simulink model "mech_robot_vr"  (Simulink 7.1)
settings: Solver=ode15s  StartTime=0.0  StopTime=1  RelTol=1e-3  AbsTol=1e-4
PreLoadFcn:
  | load mech_robot_images;mech_robot_data;
undefined symbols (not defined in the file or in its folder): Actuator, rad, s
libraries: mblibv1 x88
(part 2 of 4)

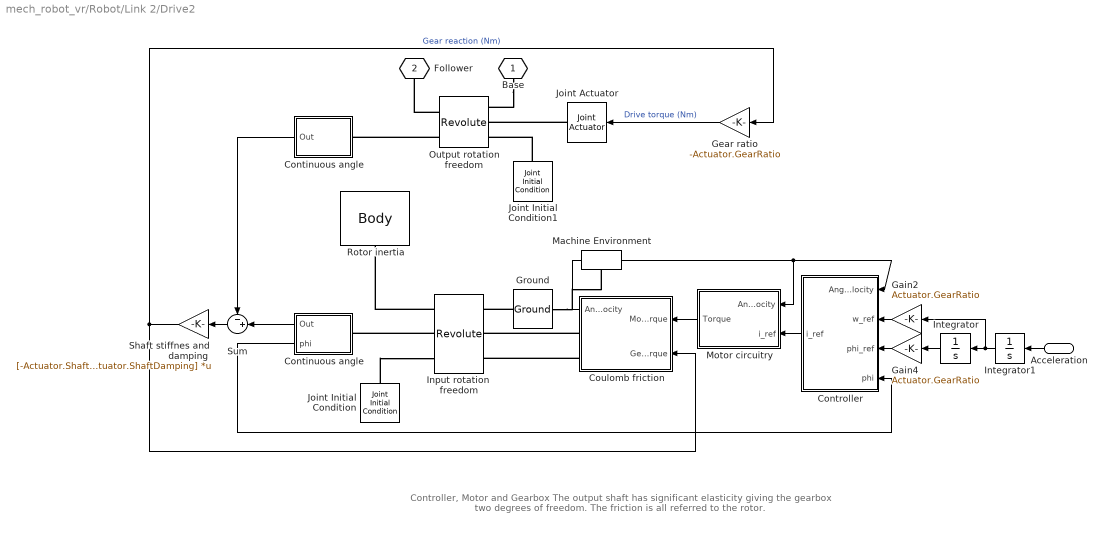
== system mech_robot_vr/Robot/Link 2/Drive2 ==
  note: Controller, Motor and Gearbox
      |
      | The output shaft has significant elasticity giving the gearbox two
      | degrees of freedom. The friction is all referred to the rotor.
  Acceleration : Inport  Orientation=left  OutDataType=sfix(16)  OutScaling=2^0
  Continuous angle : Subsystem  Orientation=left
  "Continuous angle " : Subsystem  Orientation=left
  Controller : Subsystem  Orientation=left
  Coulomb friction : Subsystem  Orientation=left  mask{peak=Actuator.PeakRatio, Rv1=Actuator.FrictionGain, Rv0=Actuator.FrictionConstant}
      mask prompts: peak "Peak ratio"; Rv1 "Friction gain (Nm.s/rad)"; Rv0 "Friction constant (Nm)"
      mask Display:
      | plot([-2 0 0 2],[-2 -1 1 2]);
      | plot([-5 5],[0 0]);
      | plot([0 0],[-5 5]);
      | plot([-0.02 -0.02],[-3 3]);
      | plot([-0.04 -0.04],[-3 3]);
      | plot([-0.06 -0.06],[-3 3]);
      | plot([-0.08 -0.08],[-3 3]);
      | plot([-0.1 -0.1],[-3 3]);
      | plot([0.02 0.02],[-3 3]);
      | plot([0.04 0.04],[-3 3]);
      | plot([0.06 0.06],[-3 3]);
      | plot([0.08 0.08],[-3 3]);
      | plot([0.1 0.1],[-3 3]);
      | plot([-2 0],[-2.03 -1.03]);
      | plot([-2 0],[-2.06 -1.06]);
      | plot([-2 0],[-2.09 -1.09]);
      | plot([-2 0],[-2.12 -1.21]);
      | plot([-2 0],[-1.97 -0.97]);
      | plot([-2 0],[-1.94 -0.94]);
      | plot([-2 0],[-1.91 -0.91]);
      | plot([-2 0],[-1.88 -0.88]);
      | 
      | plot([2 0],[2.03 1.03]);
      | plot([2 0],[2.06 1.06]);
      | plot([2 0],[2.09 1.09]);
      | plot([2 0],[2.12 1.21]);
      | plot([2 0],[1.97 0.97]);
      | plot([2 0],[1.94 0.94]);
      | plot([2 0],[1.91 0.91]);
      | plot([2 0],[1.88 0.88]);
  Gain2 : Gain  Orientation=left  Gain=Actuator.GearRatio  ParameterDataType=sfix(16)  ParameterScaling=2^0  OutDataType=sfix(16)  OutScaling=2^0  SaturateOnIntegerOverflow=on  OutDataTypeStr=Inherit: Same as input  ParamDataTypeStr=Inherit: Same as input
  Gain4 : Gain  Orientation=left  Gain=Actuator.GearRatio  ParameterDataType=sfix(16)  ParameterScaling=2^0  OutDataType=sfix(16)  OutScaling=2^0  SaturateOnIntegerOverflow=on  OutDataTypeStr=Inherit: Same as input  ParamDataTypeStr=Inherit: Same as input
  Gear ratio : Gain  Orientation=left  Gain=-Actuator.GearRatio  ParameterDataType=sfix(16)  ParameterScaling=2^0  OutDataType=sfix(16)  OutScaling=2^0  SaturateOnIntegerOverflow=on  OutDataTypeStr=Inherit: Same as input  ParamDataTypeStr=Inherit: Same as input
  Ground : mblibv1/Bodies/Ground  Orientation=left  DialogController=MECH.DynMechDlgSource  SystemSampleTime=-1  LeftPortType=env  RightPortType=workingframe  PhysicalDomain=Mechanical  DialogClass=GroundBlock  CoordPosition=[0 0 0]  CoordPositionUnits=m  StateVectorMgrId=-1  MachineId=[0 0]  ShowEnvPort=on
  Input rotation  freedom : mblibv1/Joints/Revolute  Tag=Factory generic  Description=Mechanical Blockset  Orientation=left  DialogController=MECH.DynMechDlgSource  PhysicalDomain=mechanical  SubClassName=Unknown  LeftPortType=blob  RightPortType=blob  LConnTagsString=__newl0|SA1|SA2  RConnTagsString=__newr0|SA1|SA2  NumSAPorts=4  CutJoint=off  MarkAsCut=off  Primitives=revolute  PrimitiveProps=R1$WORLD$Actuator.Axis$revolute  DialogClass=JointBlock  R1Axis=Actuator.Axis
  Integrator : Integrator  Orientation=left  InitialCondition=q0  ZeroCross=off
  Integrator1 : Integrator  Orientation=left  ZeroCross=off
  Joint Actuator : mblibv1/Sensors &  Actuators/Joint Actuator  Orientation=left  DialogController=MECH.DynMechDlgSource  SystemSampleTime=-1  PhysicalDomain=Mechanical  PortType=blob  ActuationStyle=Force  AngleUnits=deg  ArcVelocityUnits=deg/s  ArcAccelerationUnits=deg/s^2  CoordPositionUnits=m  VelocityUnits=m/s  AccelerationUnits=m/s^2  ForceUnits=N  TorqueUnits=N-m  ActiveIO=on  Width=1  DialogClass=MechanicalActuatorBlock  Primitive=R1  ReferenceFrame=Absolute (INERTIAL)
  Joint Initial Condition : mblibv1/Sensors &  Actuators/Joint Initial Condition  Orientation=up  DialogController=MECH.DynMechDlgSource  SystemSampleTime=-1  PhysicalDomain=Mechanical  DialogClass=InitialConditionBlock  Primitive=R1  CoordPosition=q0*Actuator.GearRatio  Velocity=0.0  AngleUnits=rad  ArcVelocityUnits=deg/s  CoordPositionUnits=m  VelocityUnits=m/s  InitialConditions=P1$false$0$m$rad$0$m/s$rad/s#P2$false$0$m$rad$0$m/s$rad/s#P3$false$0$m$rad$0$m/s$rad/s#R1$true$q0*Actuator.GearRatio$m$rad$0.0$m/s$deg/s#R2$false$0$m$rad$0$m/s$rad/s#R3$false$0$m$rad$0$m/s$rad/s#S$false$0$m$rad$0$m/s$rad/s  P1PIC=0  P1VIC=0  P2PIC=0  P2VIC=0  P3PIC=0  P3VIC=0  R1PIC=q0*Actuator.GearRatio  R1VIC=0.0  R2PIC=0  R2VIC=0  R3PIC=0  R3VIC=0  SPIC=0  SVIC=0
  Joint Initial Condition1 : mblibv1/Sensors &  Actuators/Joint Initial Condition  Orientation=up  DialogController=MECH.DynMechDlgSource  SystemSampleTime=-1  PhysicalDomain=Mechanical  DialogClass=InitialConditionBlock  Primitive=R1  CoordPosition=q0  Velocity=0.0  AngleUnits=rad  ArcVelocityUnits=deg/s  CoordPositionUnits=m  VelocityUnits=m/s  InitialConditions=P1$false$0$m$rad$0$m/s$rad/s#P2$false$0$m$rad$0$m/s$rad/s#P3$false$0$m$rad$0$m/s$rad/s#R1$true$q0$m$rad$0.0$m/s$deg/s#R2$false$0$m$rad$0$m/s$rad/s#R3$false$0$m$rad$0$m/s$rad/s#S$false$0$m$rad$0$m/s$rad/s  P1PIC=0  P1VIC=0  P2PIC=0  P2VIC=0  P3PIC=0  P3VIC=0  R1PIC=q0  R1VIC=0.0  R2PIC=0  R2VIC=0  R3PIC=0  R3VIC=0  SPIC=0  SVIC=0
  Machine Environment : mblibv1/Bodies/Machine Environment  Tag=Factory ground  Orientation=down  DialogController=MECH.DialogSource  SystemSampleTime=-1  PortType=env  PhysicalDomain=Mechanical  DialogTemplateClass=MECH.MachineEnvironment  SyncWhenCopied=off  Gravity=[0 -9.81 0]  GravityUnits=m/s^2  GravityAsSignal=off  Dimensionality=3D Only  AnalysisType=Forward dynamics  LinearAssemblyTolerance=1e-3  LinearAssemblyToleranceUnits=m  AngularAssemblyTolerance=1e-3  AngularAssemblyToleranceUnits=rad  ConstraintSolverType=Stabilizing  ConstraintRelTolerance=1e-4  ConstraintAbsTolerance=1e-4  UseRobustSingularityHandling=off  RedundancyAnalysisToleranceType=Automatically select tolerance  RedundancyAnalysisTolerance=1e-14  StatePerturbationType=Fixed  PerturbationSize=1e-5  VisualizeMachine=on
  Motor circuitry : Subsystem  Orientation=left  mask{Ri=10, Ra=250, Rd1=100, Rd2=100, Rd3=100, Rd4=100, Rp1=200, Rp2=50, k=Actuator.MotorGain, d=Actuator.MotorDamping, w=Actuator.MotorConstant}
      mask prompts: Ri "Ri (Ohms)"; Ra "Ra (Ohms)"; Rd1 "Rd1 (Ohms)"; Rd2 "Rd2 (Ohms)"; Rd3 "Rd3 (Ohms)"; Rd4 "Rd4 (Ohms)"; Rp1 "Rp1 (Ohms)"; Rp2 "Rp2 (Ohms)"; k "Motor gain (Nm/A)"; d "Motor damping"; w "Motor time constant"
      mask Display: plot(-140,-140,140,140,2*[-30,-30,0,-30,-30,-55]+25,(2*[20,0,20,41,20,20]+8),[0,0]+25,(2*[0,40]+8),2*[37.5,0]+25,(2*[20,20]+8),2*[10,10,0]+25,(1*[-15,6,20]+12),1*[-65,-65,-20,-20,40,40,85,85,85,40,40,-20,-20],1*[48,-20,-20,-10,-10,-20,-20,48,-20,-20,-30,-30,-20])
  Output rotation freedom : mblibv1/Joints/Revolute  Tag=Factory generic  Description=Mechanical Blockset  Orientation=left  DialogController=MECH.DynMechDlgSource  PhysicalDomain=mechanical  SubClassName=Unknown  LeftPortType=blob  RightPortType=blob  LConnTagsString=__newl0|SA1|SA2  RConnTagsString=__newr0|SA1  NumSAPorts=3  CutJoint=off  MarkAsCut=off  Primitives=revolute  PrimitiveProps=R1$WORLD$Actuator.Axis$revolute  DialogClass=JointBlock  R1Axis=Actuator.Axis
  Rotor inertia : mblibv1/Bodies/Body  Tag=Factory generic  Description=Mechanical Blockset  Orientation=up  DialogController=MECH.DynMechDlgSource  PhysicalDomain=mechanical  SubClassName=Unknown  LeftPortType=workingframe  RightPortType=workingframe  LConnTagsString=CS1  DialogClass=MechanicalBodyBlock  Mass=0.5  MassUnits=kg  InertiaUnits=kg*m^2  Inertia=Actuator.MotorInertia*eye(3)  Shape=Cylinder  ShapeDims=[1 1]  ShapeUnits=m  ShapeUse=false  Density=1  DensityUnits=kg/m^3  DensityUse=false  GraphicsMode=1  BodyColor=[0.5 0.5 0.5]  GraphicsObj=[]  AttachedToCS=1  CG=Left$CG$[0 0 0]$CS1$CS1$m$[0 0 0]$Euler X-Y-Z$deg$WORLD$false  WorkingFrames=Left$CS1$[0 0 0]$ADJOINING$ADJOINING$m$[0 0 0]$Euler X-Y-Z$deg$WORLD$true  CGPos=[0 0 0]  CGRot=[0 0 0]  CS0Pos=[]  CS0Rot=[]  CS1Pos=[0 0 0]  CS1Rot=[0 0 0]  CS2Pos=[]  CS2Rot=[]  CS3Pos=[]  CS3Rot=[]  CS4Pos=[]  CS4Rot=[]  CS5Pos=[]  CS5Rot=[]  CS6Pos=[]  CS6Rot=[]  CS7Pos=[]  CS7Rot=[]  CS8Pos=[]  CS8Rot=[]  CS9Pos=[]  CS9Rot=[]  CS10Pos=[]  CS10Rot=[]  CS11Pos=[]  CS11Rot=[]  CS12Pos=[]  CS12Rot=[]  CS13Pos=[]  CS13Rot=[]  CS14Pos=[]  CS14Rot=[]  CS15Pos=[]  CS15Rot=[]  CS16Pos=[]  CS16Rot=[]  CS17Pos=[]  CS17Rot=[]  CS18Pos=[]  CS18Rot=[]  CS19Pos=[]  CS19Rot=[]  CS20Pos=[]  CS20Rot=[]
  Shaft stiffnes and damping : Gain  Orientation=left  Gain=[-Actuator.ShaftStiffness -Actuator.ShaftDamping]  Multiplication=Matrix(K*u)  ParameterDataType=sfix(16)  ParameterScaling=2^0  OutDataType=sfix(16)  OutScaling=2^0  SaturateOnIntegerOverflow=on  OutDataTypeStr=Inherit: Same as input  ParamDataTypeStr=Inherit: Same as input
  Sum : Sum  Orientation=left  Inputs=-+|  OutDataType=sfix(16)  OutScaling=2^0  SaturateOnIntegerOverflow=on  InputSameDT=on  OutDataTypeStr=Inherit: Same as first input
  Base : PMIOPort  Tag=PMCPort  Orientation=down  Port=1  Side=Left
  Follower : PMIOPort  Tag=PMCPort  Orientation=down  Port=2  Side=Right
  wires:
  Coulomb friction/1(Angular velocity) -> Controller/1(Angular velocity), Motor circuitry/1(Angular velocity)
  Gear ratio/1 -> Joint Actuator/1  "Drive torque (Nm)"
  Integrator/1 -> Gain4/1
  Acceleration/1 -> Integrator1/1
  "Continuous angle "/1("Out ") -> Sum/1
  Gain2/1 -> Controller/2(w_ref)
  Gain4/1 -> Controller/3(phi_ref)
  Motor circuitry/1(Torque) -> Coulomb friction/1(Motor torque)
  Sum/1 -> Shaft stiffnes and damping/1
  Continuous angle/1(Out) -> Sum/2
  Continuous angle/2(phi) -> Controller/4(phi)
  Shaft stiffnes and damping/1 -> Gear ratio/1, Coulomb friction/2(Gear torque)  "Gear reaction (Nm)"
  Integrator1/1 -> Integrator/1, Gain2/1
  Controller/1(i_ref) -> Motor circuitry/2(i_ref)
  connections:
  Base/RConn1 -- Output rotation freedom/LConn1
  Output rotation freedom/RConn1 -- Follower/RConn1
  Output rotation freedom/RConn2 -- "Continuous angle "/LConn1
  Coulomb friction/RConn1 -- Input rotation  freedom/LConn2
  Coulomb friction/RConn2 -- Input rotation  freedom/LConn3
  Input rotation  freedom/RConn1 -- Rotor inertia/LConn1
  Input rotation  freedom/RConn2 -- Continuous angle/LConn1
  Ground/RConn1 -- Input rotation  freedom/LConn1
  Joint Initial Condition1/RConn1 -- Output rotation freedom/LConn3
  Joint Actuator/RConn1 -- Output rotation freedom/LConn2
  Joint Initial Condition/RConn1 -- Input rotation  freedom/RConn3
  Ground/LConn1 -- Machine Environment/RConn1

== system mech_robot_vr/Robot/Link 2/Subsystem ==
  Clock1 : Clock
      settings: Decimation=10
  Trajectory 2 : Lookup  InputValues="[0    0.1000    0.1000    1.1000    1.1000    1.2000    1.2000    1.3000]"  Table="[-15   -15     0     0    15    15     0     0]"  OutDataType=sfix(16)  OutScaling=2^0  SaturateOnIntegerOverflow=on
  Acceleration2 : Outport  OutDataType=sfix(16)  OutScaling=2^0
  wires:
  Clock1/1 -> Trajectory 2/1
  Trajectory 2/1 -> Acceleration2/1

== system mech_robot_vr/Robot/Link3/Acceleration3 ==
  Clock5 : Clock
      settings: Decimation=10
  Trajectory 3 : Lookup  InputValues="[0    0.1500    0.1500    0.6000    0.6000    0.9000    0.9000    1.2000    1.2000    1.3000]"  Table="[30.0000   30.0000  -21.5600  -21.5600         0         0   17.3300   17.3300         0         0]"  OutDataType=sfix(16)  OutScaling=2^0  SaturateOnIntegerOverflow=on
  Acceleration3 : Outport  OutDataType=sfix(16)  OutScaling=2^0
  wires:
  Clock5/1 -> Trajectory 3/1
  Trajectory 3/1 -> Acceleration3/1

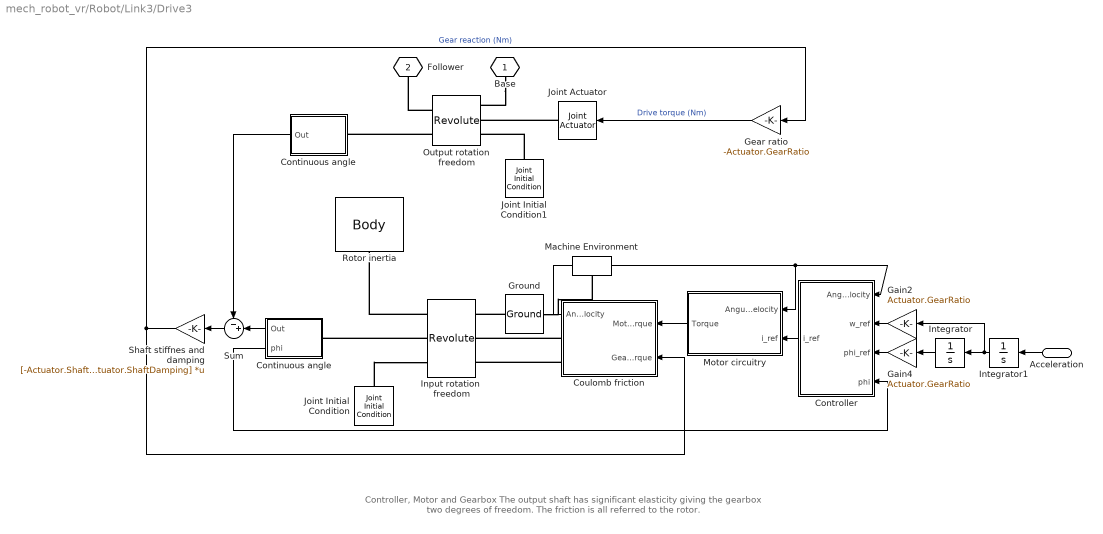
== system mech_robot_vr/Robot/Link3/Drive3 ==
  note: Controller, Motor and Gearbox
      |
      | The output shaft has significant elasticity giving the gearbox two
      | degrees of freedom. The friction is all referred to the rotor.
  Acceleration : Inport  Orientation=left  OutDataType=sfix(16)  OutScaling=2^0
  Continuous angle : Subsystem  Orientation=left
  "Continuous angle " : Subsystem  Orientation=left
  Controller : Subsystem  Orientation=left
  Coulomb friction : Subsystem  Orientation=left  mask{peak=Actuator.PeakRatio, Rv1=Actuator.FrictionGain, Rv0=Actuator.FrictionConstant}
      mask prompts: peak "Peak ratio"; Rv1 "Friction gain (Nm.s/rad)"; Rv0 "Friction constant (Nm)"
      mask Display:
      | plot([-2 0 0 2],[-2 -1 1 2]);
      | plot([-5 5],[0 0]);
      | plot([0 0],[-5 5]);
      | plot([-0.02 -0.02],[-3 3]);
      | plot([-0.04 -0.04],[-3 3]);
      | plot([-0.06 -0.06],[-3 3]);
      | plot([-0.08 -0.08],[-3 3]);
      | plot([-0.1 -0.1],[-3 3]);
      | plot([0.02 0.02],[-3 3]);
      | plot([0.04 0.04],[-3 3]);
      | plot([0.06 0.06],[-3 3]);
      | plot([0.08 0.08],[-3 3]);
      | plot([0.1 0.1],[-3 3]);
      | plot([-2 0],[-2.03 -1.03]);
      | plot([-2 0],[-2.06 -1.06]);
      | plot([-2 0],[-2.09 -1.09]);
      | plot([-2 0],[-2.12 -1.21]);
      | plot([-2 0],[-1.97 -0.97]);
      | plot([-2 0],[-1.94 -0.94]);
      | plot([-2 0],[-1.91 -0.91]);
      | plot([-2 0],[-1.88 -0.88]);
      | 
      | plot([2 0],[2.03 1.03]);
      | plot([2 0],[2.06 1.06]);
      | plot([2 0],[2.09 1.09]);
      | plot([2 0],[2.12 1.21]);
      | plot([2 0],[1.97 0.97]);
      | plot([2 0],[1.94 0.94]);
      | plot([2 0],[1.91 0.91]);
      | plot([2 0],[1.88 0.88]);
  Gain2 : Gain  Orientation=left  Gain=Actuator.GearRatio  ParameterDataType=sfix(16)  ParameterScaling=2^0  OutDataType=sfix(16)  OutScaling=2^0  SaturateOnIntegerOverflow=on  OutDataTypeStr=Inherit: Same as input  ParamDataTypeStr=Inherit: Same as input
  Gain4 : Gain  Orientation=left  Gain=Actuator.GearRatio  ParameterDataType=sfix(16)  ParameterScaling=2^0  OutDataType=sfix(16)  OutScaling=2^0  SaturateOnIntegerOverflow=on  OutDataTypeStr=Inherit: Same as input  ParamDataTypeStr=Inherit: Same as input
  Gear ratio : Gain  Orientation=left  Gain=-Actuator.GearRatio  ParameterDataType=sfix(16)  ParameterScaling=2^0  OutDataType=sfix(16)  OutScaling=2^0  SaturateOnIntegerOverflow=on  OutDataTypeStr=Inherit: Same as input  ParamDataTypeStr=Inherit: Same as input
  Ground : mblibv1/Bodies/Ground  Orientation=left  DialogController=MECH.DynMechDlgSource  SystemSampleTime=-1  LeftPortType=env  RightPortType=workingframe  PhysicalDomain=Mechanical  DialogClass=GroundBlock  CoordPosition=[0 0 0]  CoordPositionUnits=m  StateVectorMgrId=-1  MachineId=[0 0]  ShowEnvPort=on
  Input rotation  freedom : mblibv1/Joints/Revolute  Tag=Factory generic  Description=Mechanical Blockset  Orientation=left  DialogController=MECH.DynMechDlgSource  PhysicalDomain=mechanical  SubClassName=Unknown  LeftPortType=blob  RightPortType=blob  LConnTagsString=__newl0|SA1|SA2  RConnTagsString=__newr0|SA1|SA2  NumSAPorts=4  CutJoint=off  MarkAsCut=off  Primitives=revolute  PrimitiveProps=R1$WORLD$Actuator.Axis$revolute  DialogClass=JointBlock  R1Axis=Actuator.Axis
  Integrator : Integrator  Orientation=left  InitialCondition=q0  ZeroCross=off
  Integrator1 : Integrator  Orientation=left  ZeroCross=off
  Joint Actuator : mblibv1/Sensors &  Actuators/Joint Actuator  Orientation=left  DialogController=MECH.DynMechDlgSource  SystemSampleTime=-1  PhysicalDomain=Mechanical  PortType=blob  ActuationStyle=Force  AngleUnits=deg  ArcVelocityUnits=deg/s  ArcAccelerationUnits=deg/s^2  CoordPositionUnits=m  VelocityUnits=m/s  AccelerationUnits=m/s^2  ForceUnits=N  TorqueUnits=N-m  ActiveIO=on  Width=1  DialogClass=MechanicalActuatorBlock  Primitive=R1  ReferenceFrame=Absolute (INERTIAL)
  Joint Initial Condition : mblibv1/Sensors &  Actuators/Joint Initial Condition  Orientation=up  DialogController=MECH.DynMechDlgSource  SystemSampleTime=-1  PhysicalDomain=Mechanical  DialogClass=InitialConditionBlock  Primitive=R1  CoordPosition=q0*Actuator.GearRatio  Velocity=0.0  AngleUnits=rad  ArcVelocityUnits=deg/s  CoordPositionUnits=m  VelocityUnits=m/s  InitialConditions=P1$false$0$m$rad$0$m/s$rad/s#P2$false$0$m$rad$0$m/s$rad/s#P3$false$0$m$rad$0$m/s$rad/s#R1$true$q0*Actuator.GearRatio$m$rad$0.0$m/s$deg/s#R2$false$0$m$rad$0$m/s$rad/s#R3$false$0$m$rad$0$m/s$rad/s#S$false$0$m$rad$0$m/s$rad/s  P1PIC=0  P1VIC=0  P2PIC=0  P2VIC=0  P3PIC=0  P3VIC=0  R1PIC=q0*Actuator.GearRatio  R1VIC=0.0  R2PIC=0  R2VIC=0  R3PIC=0  R3VIC=0  SPIC=0  SVIC=0
  Joint Initial Condition1 : mblibv1/Sensors &  Actuators/Joint Initial Condition  Orientation=up  DialogController=MECH.DynMechDlgSource  SystemSampleTime=-1  PhysicalDomain=Mechanical  DialogClass=InitialConditionBlock  Primitive=R1  CoordPosition=q0  Velocity=0.0  AngleUnits=rad  ArcVelocityUnits=deg/s  CoordPositionUnits=m  VelocityUnits=m/s  InitialConditions=P1$false$0$m$rad$0$m/s$rad/s#P2$false$0$m$rad$0$m/s$rad/s#P3$false$0$m$rad$0$m/s$rad/s#R1$true$q0$m$rad$0.0$m/s$deg/s#R2$false$0$m$rad$0$m/s$rad/s#R3$false$0$m$rad$0$m/s$rad/s#S$false$0$m$rad$0$m/s$rad/s  P1PIC=0  P1VIC=0  P2PIC=0  P2VIC=0  P3PIC=0  P3VIC=0  R1PIC=q0  R1VIC=0.0  R2PIC=0  R2VIC=0  R3PIC=0  R3VIC=0  SPIC=0  SVIC=0
  Machine Environment : mblibv1/Bodies/Machine Environment  Tag=Factory ground  Orientation=down  DialogController=MECH.DialogSource  SystemSampleTime=-1  PortType=env  PhysicalDomain=Mechanical  DialogTemplateClass=MECH.MachineEnvironment  SyncWhenCopied=off  Gravity=[0 -9.81 0]  GravityUnits=m/s^2  GravityAsSignal=off  Dimensionality=3D Only  AnalysisType=Forward dynamics  LinearAssemblyTolerance=1e-3  LinearAssemblyToleranceUnits=m  AngularAssemblyTolerance=1e-3  AngularAssemblyToleranceUnits=rad  ConstraintSolverType=Stabilizing  ConstraintRelTolerance=1e-4  ConstraintAbsTolerance=1e-4  UseRobustSingularityHandling=off  RedundancyAnalysisToleranceType=Automatically select tolerance  RedundancyAnalysisTolerance=1e-14  StatePerturbationType=Fixed  PerturbationSize=1e-5  VisualizeMachine=on
  Motor circuitry : Subsystem  Orientation=left  mask{Ri=10, Ra=250, Rd1=100, Rd2=100, Rd3=100, Rd4=100, Rp1=200, Rp2=50, k=Actuator.MotorGain, d=Actuator.MotorDamping, w=Actuator.MotorConstant}
      mask prompts: Ri "Ri (Ohms)"; Ra "Ra (Ohms)"; Rd1 "Rd1 (Ohms)"; Rd2 "Rd2 (Ohms)"; Rd3 "Rd3 (Ohms)"; Rd4 "Rd4 (Ohms)"; Rp1 "Rp1 (Ohms)"; Rp2 "Rp2 (Ohms)"; k "Motor gain (Nm/A)"; d "Motor damping"; w "Motor time constant"
      mask Display: plot(-140,-140,140,140,2*[-30,-30,0,-30,-30,-55]+25,(2*[20,0,20,41,20,20]+8),[0,0]+25,(2*[0,40]+8),2*[37.5,0]+25,(2*[20,20]+8),2*[10,10,0]+25,(1*[-15,6,20]+12),1*[-65,-65,-20,-20,40,40,85,85,85,40,40,-20,-20],1*[48,-20,-20,-10,-10,-20,-20,48,-20,-20,-30,-30,-20])
  Output rotation freedom : mblibv1/Joints/Revolute  Tag=Factory generic  Description=Mechanical Blockset  Orientation=left  DialogController=MECH.DynMechDlgSource  PhysicalDomain=mechanical  SubClassName=Unknown  LeftPortType=blob  RightPortType=blob  LConnTagsString=__newl0|SA1|SA2  RConnTagsString=__newr0|SA1  NumSAPorts=3  CutJoint=off  MarkAsCut=off  Primitives=revolute  PrimitiveProps=R1$WORLD$Actuator.Axis$revolute  DialogClass=JointBlock  R1Axis=Actuator.Axis
  Rotor inertia : mblibv1/Bodies/Body  Tag=Factory generic  Description=Mechanical Blockset  Orientation=up  DialogController=MECH.DynMechDlgSource  PhysicalDomain=mechanical  SubClassName=Unknown  LeftPortType=workingframe  RightPortType=workingframe  LConnTagsString=CS1  DialogClass=MechanicalBodyBlock  Mass=0.5  MassUnits=kg  InertiaUnits=kg*m^2  Inertia=Actuator.MotorInertia*eye(3)  Shape=Cylinder  ShapeDims=[1 1]  ShapeUnits=m  ShapeUse=false  Density=1  DensityUnits=kg/m^3  DensityUse=false  GraphicsMode=1  BodyColor=[0.5 0.5 0.5]  GraphicsObj=[]  AttachedToCS=1  CG=Left$CG$[0 0 0]$CS1$CS1$m$[0 0 0]$Euler X-Y-Z$deg$WORLD$false  WorkingFrames=Left$CS1$[0 0 0]$ADJOINING$ADJOINING$m$[0 0 0]$Euler X-Y-Z$deg$WORLD$true  CGPos=[0 0 0]  CGRot=[0 0 0]  CS0Pos=[]  CS0Rot=[]  CS1Pos=[0 0 0]  CS1Rot=[0 0 0]  CS2Pos=[]  CS2Rot=[]  CS3Pos=[]  CS3Rot=[]  CS4Pos=[]  CS4Rot=[]  CS5Pos=[]  CS5Rot=[]  CS6Pos=[]  CS6Rot=[]  CS7Pos=[]  CS7Rot=[]  CS8Pos=[]  CS8Rot=[]  CS9Pos=[]  CS9Rot=[]  CS10Pos=[]  CS10Rot=[]  CS11Pos=[]  CS11Rot=[]  CS12Pos=[]  CS12Rot=[]  CS13Pos=[]  CS13Rot=[]  CS14Pos=[]  CS14Rot=[]  CS15Pos=[]  CS15Rot=[]  CS16Pos=[]  CS16Rot=[]  CS17Pos=[]  CS17Rot=[]  CS18Pos=[]  CS18Rot=[]  CS19Pos=[]  CS19Rot=[]  CS20Pos=[]  CS20Rot=[]
  Shaft stiffnes and damping : Gain  Orientation=left  Gain=[-Actuator.ShaftStiffness -Actuator.ShaftDamping]  Multiplication=Matrix(K*u)  ParameterDataType=sfix(16)  ParameterScaling=2^0  OutDataType=sfix(16)  OutScaling=2^0  SaturateOnIntegerOverflow=on  OutDataTypeStr=Inherit: Same as input  ParamDataTypeStr=Inherit: Same as input
  Sum : Sum  Orientation=left  Inputs=-+|  OutDataType=sfix(16)  OutScaling=2^0  SaturateOnIntegerOverflow=on  InputSameDT=on  OutDataTypeStr=Inherit: Same as first input
  Base : PMIOPort  Tag=PMCPort  Orientation=down  Port=1  Side=Left
  Follower : PMIOPort  Tag=PMCPort  Orientation=down  Port=2  Side=Right
  wires:
  Coulomb friction/1(Angular velocity) -> Controller/1(Angular velocity), Motor circuitry/1(Angular velocity)
  Gear ratio/1 -> Joint Actuator/1  "Drive torque (Nm)"
  Integrator/1 -> Gain4/1
  Acceleration/1 -> Integrator1/1
  "Continuous angle "/1("Out ") -> Sum/1
  Gain2/1 -> Controller/2(w_ref)
  Gain4/1 -> Controller/3(phi_ref)
  Controller/1(i_ref) -> Motor circuitry/2(i_ref)
  Motor circuitry/1(Torque) -> Coulomb friction/1(Motor torque)
  Sum/1 -> Shaft stiffnes and damping/1
  Continuous angle/1(Out) -> Sum/2
  Continuous angle/2(phi) -> Controller/4(phi)
  Integrator1/1 -> Integrator/1, Gain2/1
  Shaft stiffnes and damping/1 -> Gear ratio/1, Coulomb friction/2(Gear torque)  "Gear reaction (Nm)"
  connections:
  Base/RConn1 -- Output rotation freedom/LConn1
  Output rotation freedom/RConn1 -- Follower/RConn1
  Output rotation freedom/RConn2 -- "Continuous angle "/LConn1
  Coulomb friction/RConn1 -- Input rotation  freedom/LConn2
  Coulomb friction/RConn2 -- Input rotation  freedom/LConn3
  Input rotation  freedom/RConn1 -- Rotor inertia/LConn1
  Input rotation  freedom/RConn2 -- Continuous angle/LConn1
  Ground/RConn1 -- Input rotation  freedom/LConn1
  Joint Initial Condition1/RConn1 -- Output rotation freedom/LConn3
  Joint Actuator/RConn1 -- Output rotation freedom/LConn2
  Joint Initial Condition/RConn1 -- Input rotation  freedom/RConn3
  Ground/LConn1 -- Machine Environment/RConn1

== system mech_robot_vr/Robot/Link4/Drive4 ==
  note: Controller, motor and ideal gear
      | No elasticity is modelled in this gear. All friction is referred
      | to the rotor.
  Acceleration : Inport  Orientation=left  OutDataType=sfix(16)  OutScaling=2^0
  Continuous angle : Subsystem
  Controller : Subsystem  Orientation=left
  Coulomb friction : Subsystem  Orientation=left  mask{peak=Actuator.PeakRatio, Rv1=Actuator.FrictionGain, Rv0=Actuator.FrictionConstant}
      mask prompts: peak "Peak ratio"; Rv1 "Friction gain (Nm.s/rad)"; Rv0 "Friction constant (Nm)"
      mask Display:
      | plot([-2 0 0 2],[-2 -1 1 2]);
      | plot([-5 5],[0 0]);
      | plot([0 0],[-5 5]);
      | plot([-0.02 -0.02],[-3 3]);
      | plot([-0.04 -0.04],[-3 3]);
      | plot([-0.06 -0.06],[-3 3]);
      | plot([-0.08 -0.08],[-3 3]);
      | plot([-0.1 -0.1],[-3 3]);
      | plot([0.02 0.02],[-3 3]);
      | plot([0.04 0.04],[-3 3]);
      | plot([0.06 0.06],[-3 3]);
      | plot([0.08 0.08],[-3 3]);
      | plot([0.1 0.1],[-3 3]);
      | plot([-2 0],[-2.03 -1.03]);
      | plot([-2 0],[-2.06 -1.06]);
      | plot([-2 0],[-2.09 -1.09]);
      | plot([-2 0],[-2.12 -1.21]);
      | plot([-2 0],[-1.97 -0.97]);
      | plot([-2 0],[-1.94 -0.94]);
      | plot([-2 0],[-1.91 -0.91]);
      | plot([-2 0],[-1.88 -0.88]);
      | 
      | plot([2 0],[2.03 1.03]);
      | plot([2 0],[2.06 1.06]);
      | plot([2 0],[2.09 1.09]);
      | plot([2 0],[2.12 1.21]);
      | plot([2 0],[1.97 0.97]);
      | plot([2 0],[1.94 0.94]);
      | plot([2 0],[1.91 0.91]);
      | plot([2 0],[1.88 0.88]);
  Gain2 : Gain  Orientation=left  Gain=Actuator.GearRatio  ParameterDataType=sfix(16)  ParameterScaling=2^0  OutDataType=sfix(16)  OutScaling=2^0  SaturateOnIntegerOverflow=on  OutDataTypeStr=Inherit: Same as input  ParamDataTypeStr=Inherit: Same as input
  Gain4 : Gain  Orientation=left  Gain=Actuator.GearRatio  ParameterDataType=sfix(16)  ParameterScaling=2^0  OutDataType=sfix(16)  OutScaling=2^0  SaturateOnIntegerOverflow=on  OutDataTypeStr=Inherit: Same as input  ParamDataTypeStr=Inherit: Same as input
  Ideal gear : Subsystem  Orientation=left  mask{ig=Actuator.GearRatio, Axis=Actuator.Axis, q0=q0}
      mask prompts: ig "Gear ratio"; Axis "Rotation axis"; q0 "Initial angle (rad)"
      mask init:
      | Vector = null(Axis(:)')*[1;0];
      | Null = cross(Axis,Vector);
      | T = [Axis(:),Vector(:),Null(:)];
      | Vector = (1e-2 - 1e-2/ig)*Vector;
  Integrator2 : Integrator  Orientation=left  InitialCondition=q0  ZeroCross=off
  Integrator3 : Integrator  Orientation=left  ZeroCross=off
  Motor circuitry : Subsystem  Orientation=left  mask{Ri=10, Ra=250, Rd1=100, Rd2=100, Rd3=100, Rd4=100, Rp1=200, Rp2=50, k=Actuator.MotorGain, d=Actuator.MotorDamping, w=Actuator.MotorConstant}
      mask prompts: Ri "Ri (Ohms)"; Ra "Ra (Ohms)"; Rd1 "Rd1 (Ohms)"; Rd2 "Rd2 (Ohms)"; Rd3 "Rd3 (Ohms)"; Rd4 "Rd4 (Ohms)"; Rp1 "Rp1 (Ohms)"; Rp2 "Rp2 (Ohms)"; k "Motor gain (Nm/A)"; d "Motor damping"; w "Motor time constant"
      mask Display: plot(-140,-140,140,140,2*[-30,-30,0,-30,-30,-55]+25,(2*[20,0,20,41,20,20]+8),[0,0]+25,(2*[0,40]+8),2*[37.5,0]+25,(2*[20,20]+8),2*[10,10,0]+25,(1*[-15,6,20]+12),1*[-65,-65,-20,-20,40,40,85,85,85,40,40,-20,-20],1*[48,-20,-20,-10,-10,-20,-20,48,-20,-20,-30,-30,-20])
  Base : PMIOPort  Tag=PMCPort  Orientation=left  Port=1  Side=Left
  Follower : PMIOPort  Tag=PMCPort  Port=2  Side=Right
  wires:
  Integrator2/1 -> Gain4/1
  Acceleration/1 -> Integrator3/1
  Gain2/1 -> Controller/3(w_ref)
  Gain4/1 -> Controller/4(phi_ref)
  Controller/1(i_ref) -> Motor circuitry/2(i_ref)
  Motor circuitry/1(Torque) -> Coulomb friction/1(Motor torque)
  Integrator3/1 -> Integrator2/1, Gain2/1
  Coulomb friction/1(phi) -> Continuous angle/2(phi)
  Coulomb friction/2(Angular velocity) -> Continuous angle/1(Angular velocity)
  Continuous angle/1("phi ") -> Controller/2(phi)
  Continuous angle/2("Angular velocity ") -> Controller/1(Angular velocity), Motor circuitry/1(Angular velocity)
  connections:
  Ideal gear/RConn1 -- Follower/RConn1
  Coulomb friction/RConn1 -- Ideal gear/LConn2
  Coulomb friction/RConn2 -- Ideal gear/LConn3
  Base/RConn1 -- Ideal gear/LConn1

== system mech_robot_vr/Robot/Link4/Subsystem1 ==
  Clock4 : Clock
      settings: Decimation=10
  Trajectory 4 : Lookup  InputValues="[ 0    0.0400    0.0400    0.5400    0.5400    0.6300    0.6300    1.1400    1.1400    1.2000    1.2000 1.3]"  Table="[-80.0000  -80.0000         0         0   71.1100   71.1100         0         0  -53.3300  -53.3300         0 0]"  OutDataType=sfix(16)  OutScaling=2^0  SaturateOnIntegerOverflow=on
  Acceleration4 : Outport  OutDataType=sfix(16)  OutScaling=2^0
  wires:
  Clock4/1 -> Trajectory 4/1
  Trajectory 4/1 -> Acceleration4/1

== system mech_robot_vr/Robot/Link5/Drive5 ==
  note: Controller, motor and ideal gear
      | No elasticity is modelled in this gear. All friction is referred
      | to the rotor.
  Acceleration : Inport  Orientation=left  OutDataType=sfix(16)  OutScaling=2^0
  Continuous angle : Subsystem
  Controller : Subsystem  Orientation=left
  Coulomb friction : Subsystem  Orientation=left  mask{peak=Actuator.PeakRatio, Rv1=Actuator.FrictionGain, Rv0=Actuator.FrictionConstant}
      mask prompts: peak "Peak ratio"; Rv1 "Friction gain (Nm.s/rad)"; Rv0 "Friction constant (Nm)"
      mask Display:
      | plot([-2 0 0 2],[-2 -1 1 2]);
      | plot([-5 5],[0 0]);
      | plot([0 0],[-5 5]);
      | plot([-0.02 -0.02],[-3 3]);
      | plot([-0.04 -0.04],[-3 3]);
      | plot([-0.06 -0.06],[-3 3]);
      | plot([-0.08 -0.08],[-3 3]);
      | plot([-0.1 -0.1],[-3 3]);
      | plot([0.02 0.02],[-3 3]);
      | plot([0.04 0.04],[-3 3]);
      | plot([0.06 0.06],[-3 3]);
      | plot([0.08 0.08],[-3 3]);
      | plot([0.1 0.1],[-3 3]);
      | plot([-2 0],[-2.03 -1.03]);
      | plot([-2 0],[-2.06 -1.06]);
      | plot([-2 0],[-2.09 -1.09]);
      | plot([-2 0],[-2.12 -1.21]);
      | plot([-2 0],[-1.97 -0.97]);
      | plot([-2 0],[-1.94 -0.94]);
      | plot([-2 0],[-1.91 -0.91]);
      | plot([-2 0],[-1.88 -0.88]);
      | 
      | plot([2 0],[2.03 1.03]);
      | plot([2 0],[2.06 1.06]);
      | plot([2 0],[2.09 1.09]);
      | plot([2 0],[2.12 1.21]);
      | plot([2 0],[1.97 0.97]);
      | plot([2 0],[1.94 0.94]);
      | plot([2 0],[1.91 0.91]);
      | plot([2 0],[1.88 0.88]);
  Gain2 : Gain  Orientation=left  Gain=Actuator.GearRatio  ParameterDataType=sfix(16)  ParameterScaling=2^0  OutDataType=sfix(16)  OutScaling=2^0  SaturateOnIntegerOverflow=on  OutDataTypeStr=Inherit: Same as input  ParamDataTypeStr=Inherit: Same as input
  Gain4 : Gain  Orientation=left  Gain=Actuator.GearRatio  ParameterDataType=sfix(16)  ParameterScaling=2^0  OutDataType=sfix(16)  OutScaling=2^0  SaturateOnIntegerOverflow=on  OutDataTypeStr=Inherit: Same as input  ParamDataTypeStr=Inherit: Same as input
  Ideal gear : Subsystem  Orientation=left  mask{ig=Actuator.GearRatio, Axis=Actuator.Axis, q0=q0}
      mask prompts: ig "Gear ratio"; Axis "Rotation axis"; q0 "Initial angle (rad)"
      mask init:
      | Vector = null(Axis(:)')*[1;0];
      | Null = cross(Axis,Vector);
      | T = [Axis(:),Vector(:),Null(:)];
      | Vector = (1e-2 - 1e-2/ig)*Vector;
  Integrator2 : Integrator  Orientation=left  InitialCondition=q0  ZeroCross=off
  Integrator3 : Integrator  Orientation=left  ZeroCross=off
  Motor circuitry : Subsystem  Orientation=left  mask{Ri=10, Ra=250, Rd1=100, Rd2=100, Rd3=100, Rd4=100, Rp1=200, Rp2=50, k=Actuator.MotorGain, d=Actuator.MotorDamping, w=Actuator.MotorConstant}
      mask prompts: Ri "Ri (Ohms)"; Ra "Ra (Ohms)"; Rd1 "Rd1 (Ohms)"; Rd2 "Rd2 (Ohms)"; Rd3 "Rd3 (Ohms)"; Rd4 "Rd4 (Ohms)"; Rp1 "Rp1 (Ohms)"; Rp2 "Rp2 (Ohms)"; k "Motor gain (Nm/A)"; d "Motor damping"; w "Motor time constant"
      mask Display: plot(-140,-140,140,140,2*[-30,-30,0,-30,-30,-55]+25,(2*[20,0,20,41,20,20]+8),[0,0]+25,(2*[0,40]+8),2*[37.5,0]+25,(2*[20,20]+8),2*[10,10,0]+25,(1*[-15,6,20]+12),1*[-65,-65,-20,-20,40,40,85,85,85,40,40,-20,-20],1*[48,-20,-20,-10,-10,-20,-20,48,-20,-20,-30,-30,-20])
  Base : PMIOPort  Tag=PMCPort  Orientation=left  Port=1  Side=Left
  Follower : PMIOPort  Tag=PMCPort  Port=2  Side=Right
  wires:
  Integrator2/1 -> Gain4/1
  Acceleration/1 -> Integrator3/1
  Gain2/1 -> Controller/3(w_ref)
  Gain4/1 -> Controller/4(phi_ref)
  Motor circuitry/1(Torque) -> Coulomb friction/1(Motor torque)
  Integrator3/1 -> Integrator2/1, Gain2/1
  Coulomb friction/1(phi) -> Continuous angle/2(phi)
  Coulomb friction/2(Angular velocity) -> Continuous angle/1(Angular velocity)
  Continuous angle/1("phi ") -> Controller/2(phi)
  Continuous angle/2("Angular velocity ") -> Controller/1(Angular velocity), Motor circuitry/1(Angular velocity)
  Controller/1(i_ref) -> Motor circuitry/2(i_ref)
  connections:
  Ideal gear/RConn1 -- Follower/RConn1
  Coulomb friction/RConn1 -- Ideal gear/LConn2
  Coulomb friction/RConn2 -- Ideal gear/LConn3
  Base/RConn1 -- Ideal gear/LConn1

== system mech_robot_vr/Robot/Link5/Subsystem2 ==
  Clock3 : Clock
      settings: Decimation=10
  Trajectory 5 : Lookup  InputValues="[0    0.0400    0.0400    1.0200    1.0200    1.1400    1.1400    1.2000    1.2000    1.3000]"  Table="[105.0000  105.0000         0         0  -68.3300  -68.3300   66.6700   66.6700         0         0]"  OutDataType=sfix(16)  OutScaling=2^0  SaturateOnIntegerOverflow=on
  Acceleration5 : Outport  OutDataType=sfix(16)  OutScaling=2^0
  wires:
  Clock3/1 -> Trajectory 5/1
  Trajectory 5/1 -> Acceleration5/1

== system mech_robot_vr/Robot/Link6/Drive6 ==
  note: Controller, motor and ideal gear
      | No elasticity is modelled in this gear. All friction is referred
      | to the rotor.
  Acceleration : Inport  Orientation=left  OutDataType=sfix(16)  OutScaling=2^0
  Continuous angle : Subsystem
  Controller : Subsystem  Orientation=left
  Coulomb friction : Subsystem  Orientation=left  mask{peak=Actuator.PeakRatio, Rv1=Actuator.FrictionGain, Rv0=Actuator.FrictionConstant}
      mask prompts: peak "Peak ratio"; Rv1 "Friction gain (Nm.s/rad)"; Rv0 "Friction constant (Nm)"
      mask Display:
      | plot([-2 0 0 2],[-2 -1 1 2]);
      | plot([-5 5],[0 0]);
      | plot([0 0],[-5 5]);
      | plot([-0.02 -0.02],[-3 3]);
      | plot([-0.04 -0.04],[-3 3]);
      | plot([-0.06 -0.06],[-3 3]);
      | plot([-0.08 -0.08],[-3 3]);
      | plot([-0.1 -0.1],[-3 3]);
      | plot([0.02 0.02],[-3 3]);
      | plot([0.04 0.04],[-3 3]);
      | plot([0.06 0.06],[-3 3]);
      | plot([0.08 0.08],[-3 3]);
      | plot([0.1 0.1],[-3 3]);
      | plot([-2 0],[-2.03 -1.03]);
      | plot([-2 0],[-2.06 -1.06]);
      | plot([-2 0],[-2.09 -1.09]);
      | plot([-2 0],[-2.12 -1.21]);
      | plot([-2 0],[-1.97 -0.97]);
      | plot([-2 0],[-1.94 -0.94]);
      | plot([-2 0],[-1.91 -0.91]);
      | plot([-2 0],[-1.88 -0.88]);
      | 
      | plot([2 0],[2.03 1.03]);
      | plot([2 0],[2.06 1.06]);
      | plot([2 0],[2.09 1.09]);
      | plot([2 0],[2.12 1.21]);
      | plot([2 0],[1.97 0.97]);
      | plot([2 0],[1.94 0.94]);
      | plot([2 0],[1.91 0.91]);
      | plot([2 0],[1.88 0.88]);
  Gain2 : Gain  Orientation=left  Gain=Actuator.GearRatio  ParameterDataType=sfix(16)  ParameterScaling=2^0  OutDataType=sfix(16)  OutScaling=2^0  SaturateOnIntegerOverflow=on  OutDataTypeStr=Inherit: Same as input  ParamDataTypeStr=Inherit: Same as input
  Gain4 : Gain  Orientation=left  Gain=Actuator.GearRatio  ParameterDataType=sfix(16)  ParameterScaling=2^0  OutDataType=sfix(16)  OutScaling=2^0  SaturateOnIntegerOverflow=on  OutDataTypeStr=Inherit: Same as input  ParamDataTypeStr=Inherit: Same as input
  Ideal gear : Subsystem  Orientation=left  mask{ig=Actuator.GearRatio, Axis=Actuator.Axis, q0=q0}
      mask prompts: ig "Gear ratio"; Axis "Rotation axis"; q0 "Initial angle (rad)"
      mask init:
      | Vector = null(Axis(:)')*[1;0];
      | Null = cross(Axis,Vector);
      | T = [Axis(:),Vector(:),Null(:)];
      | Vector = (1e-2 - 1e-2/ig)*Vector;
  Integrator2 : Integrator  Orientation=left  InitialCondition=q0  ZeroCross=off
  Integrator3 : Integrator  Orientation=left  ZeroCross=off
  Motor circuitry : Subsystem  Orientation=left  mask{Ri=10, Ra=250, Rd1=100, Rd2=100, Rd3=100, Rd4=100, Rp1=200, Rp2=50, k=Actuator.MotorGain, d=Actuator.MotorDamping, w=Actuator.MotorConstant}
      mask prompts: Ri "Ri (Ohms)"; Ra "Ra (Ohms)"; Rd1 "Rd1 (Ohms)"; Rd2 "Rd2 (Ohms)"; Rd3 "Rd3 (Ohms)"; Rd4 "Rd4 (Ohms)"; Rp1 "Rp1 (Ohms)"; Rp2 "Rp2 (Ohms)"; k "Motor gain (Nm/A)"; d "Motor damping"; w "Motor time constant"
      mask Display: plot(-140,-140,140,140,2*[-30,-30,0,-30,-30,-55]+25,(2*[20,0,20,41,20,20]+8),[0,0]+25,(2*[0,40]+8),2*[37.5,0]+25,(2*[20,20]+8),2*[10,10,0]+25,(1*[-15,6,20]+12),1*[-65,-65,-20,-20,40,40,85,85,85,40,40,-20,-20],1*[48,-20,-20,-10,-10,-20,-20,48,-20,-20,-30,-30,-20])
  Base : PMIOPort  Tag=PMCPort  Orientation=left  Port=1  Side=Left
  Follower : PMIOPort  Tag=PMCPort  Port=2  Side=Right
  wires:
  Integrator2/1 -> Gain4/1
  Acceleration/1 -> Integrator3/1
  Gain2/1 -> Controller/3(w_ref)
  Gain4/1 -> Controller/4(phi_ref)
  Motor circuitry/1(Torque) -> Coulomb friction/1(Motor torque)
  Integrator3/1 -> Integrator2/1, Gain2/1
  Coulomb friction/1(phi) -> Continuous angle/2(phi)
  Coulomb friction/2(Angular velocity) -> Continuous angle/1(Angular velocity)
  Continuous angle/1("phi ") -> Controller/2(phi)
  Continuous angle/2("Angular velocity ") -> Controller/1(Angular velocity), Motor circuitry/1(Angular velocity)
  Controller/1(i_ref) -> Motor circuitry/2(i_ref)
  connections:
  Ideal gear/RConn1 -- Follower/RConn1
  Coulomb friction/RConn1 -- Ideal gear/LConn2
  Coulomb friction/RConn2 -- Ideal gear/LConn3
  Base/RConn1 -- Ideal gear/LConn1

== system mech_robot_vr/Robot/Link6/Subsystem3 ==
  Clock2 : Clock
      settings: Decimation=10
  Trajectory 6 : Lookup  InputValues="[0    0.0400    0.0400    0.5400    0.5400    0.6300    0.6300    1.1400    1.1400    1.2000    1.2000 1.3]"  Table="[-95.0000  -95.0000         0         0   84.4400   84.4400         0         0  -63.3300  -63.3300         0 0]"  OutDataType=sfix(16)  OutScaling=2^0  SaturateOnIntegerOverflow=on
  Acceleration6 : Outport  OutDataType=sfix(16)  OutScaling=2^0
  wires:
  Clock2/1 -> Trajectory 6/1
  Trajectory 6/1 -> Acceleration6/1

== system mech_robot_vr/Robot/Link 1/Drive1/Continuous angle ==
  Continuous Angle : Subsystem  Tag=Factory continuousAngle  Orientation=left  AncestorBlock=mblibv1/Utilities/Continuous Angle  mask{rad=rad, rads=rad/s}
      mask prompts: rad "Angle measured in:"; rads "Rate measured in:"
      mask help: Outputs a continuous, unbounded angle given a discontinuous, bounded angle and the angular velocity. Choose units for the angle and the angular velocity (rate).
      mask Help: web(mech_help('continuousangle'))
      mask StyleString: popup(rad|deg),popup(rad/s|deg/s)
  Demux : Demux  Orientation=left  Outputs=2
  Joint Sensor : mblibv1/Sensors &  Actuators/Joint Sensor  Orientation=left  DialogController=MECH.DynMechDlgSource  SystemSampleTime=-1  PhysicalDomain=Mechanical  PortType=blob  Muxed=on  Pose=off  Angle=on  AngleUnits=rad  ArcVelocity=on  ArcVelocityUnits=rad/s  ArcAcceleration=off  ArcAccelerationUnits=deg/s^2  CoordPosition=on  CoordPositionUnits=m  Velocity=off  VelocityUnits=m/s  Acceleration=off  AccelerationUnits=m/s^2  Quaternion=on  QuaternionDT=off  QuaternionDDT=off  QuaternionUnits=off  OutputVector=[ 1 1 ]  ActiveIO=on  Width=2  DialogClass=MechanicalSensorBlock  Primitive=R1  Force=off  ForceUnits=N  Torque=off  TorqueUnits=N-m  ReferenceFrame=Absolute (INERTIAL)  ReactionSensedSide=Base  ReactionReferenceFrame=Absolute (World)  ReactionForce=off  ReactionForceUnits=N  ReactionMoment=off  ReactionMomentUnits=N-m
  Mux : Mux  Orientation=left  Inputs=2
  In : PMIOPort  Orientation=left  Port=1  Side=Left
  Out : Outport  Orientation=left  OutDataType=sfix(16)  OutScaling=2^0
  phi : Outport  Orientation=left  Port=2  OutDataType=sfix(16)  OutScaling=2^0
  wires:
  Mux/1 -> Out/1
  Continuous Angle/1(Continuous Angle) -> Mux/1, phi/1
  Demux/2 -> Mux/2, Continuous Angle/2(Rate)
  Demux/1 -> Continuous Angle/1(Angle)
  Joint Sensor/1 -> Demux/1
  connections:
  In/RConn1 -- Joint Sensor/LConn1

== system mech_robot_vr/Robot/Link 1/Drive1/Continuous angle  ==
  Continuous Angle : mblibv1/Utilities/Continuous Angle  Tag=Factory continuousAngle  Orientation=left  SystemSampleTime=-1  rad=rad  rads=rad/s
  Demux : Demux  Orientation=left  Outputs=2
  Gain2 : Gain  Orientation=left  Gain=Actuator.GearRatio  ParameterDataType=sfix(16)  ParameterScaling=2^0  OutDataType=sfix(16)  OutScaling=2^0  SaturateOnIntegerOverflow=on  OutDataTypeStr=Inherit: Same as input  ParamDataTypeStr=Inherit: Same as input
  Joint Sensor : mblibv1/Sensors &  Actuators/Joint Sensor  Orientation=left  DialogController=MECH.DynMechDlgSource  SystemSampleTime=-1  PhysicalDomain=Mechanical  PortType=blob  Muxed=on  Pose=off  Angle=on  AngleUnits=rad  ArcVelocity=on  ArcVelocityUnits=rad/s  ArcAcceleration=off  ArcAccelerationUnits=deg/s^2  CoordPosition=on  CoordPositionUnits=m  Velocity=off  VelocityUnits=m/s  Acceleration=off  AccelerationUnits=m/s^2  Quaternion=on  QuaternionDT=off  QuaternionDDT=off  QuaternionUnits=off  OutputVector=[ 1 1 ]  ActiveIO=on  Width=2  DialogClass=MechanicalSensorBlock  Primitive=R1  Force=off  ForceUnits=N  Torque=off  TorqueUnits=N-m  ReferenceFrame=Absolute (INERTIAL)  ReactionSensedSide=Base  ReactionReferenceFrame=Absolute (World)  ReactionForce=off  ReactionForceUnits=N  ReactionMoment=off  ReactionMomentUnits=N-m
  Mux : Mux  Orientation=left  Inputs=2
  To Workspace : ToWorkspace  VariableName=Body1_D  SampleTime=-1  SaveFormat=Structure With Time
  In : PMIOPort  Orientation=left  Port=1  Side=Left
  "Out " : Outport  Orientation=left  OutDataType=sfix(16)  OutScaling=2^0
  tag scope: Body1=global
  wires:
  Joint Sensor/1 -> Demux/1
  Demux/1 -> Continuous Angle/1
  Demux/2 -> Continuous Angle/2, Mux/2
  Continuous Angle/1 -> Mux/1, [Body1], To Workspace/1
  Mux/1 -> Gain2/1
  Gain2/1 -> "Out "/1
  connections:
  In/RConn1 -- Joint Sensor/LConn1

== system mech_robot_vr/Robot/Link 1/Drive1/Controller ==
  Angular velocity : Inport  OutDataType=sfix(16)  OutScaling=2^0
  w_ref : Inport  Orientation=down  Port=2  OutDataType=sfix(16)  OutScaling=2^0
  phi_ref : Inport  Port=3  OutDataType=sfix(16)  OutScaling=2^0
  phi : Inport  Port=4  OutDataType=sfix(16)  OutScaling=2^0
  Integrator : Integrator  ZeroCross=off
  Lead filter : TransferFcn  Numerator=[340.8*9.95e-3 340.8]  Denominator=[0.56e-3 1]
  Position gain : Gain  Gain=0.3  ParameterDataType=sfix(16)  ParameterScaling=2^0  OutDataType=sfix(16)  OutScaling=2^0  SaturateOnIntegerOverflow=on  OutDataTypeStr=Inherit: Same as input  ParamDataTypeStr=Inherit: Same as input
  Rate controller : TransferFcn  Orientation=up  Numerator=[40e-3 1]  Denominator=[20.2e-3 1]
  Sum : Sum  Inputs=|+-  OutDataType=sfix(16)  OutScaling=2^0  SaturateOnIntegerOverflow=on
  Sum1 : Sum  Inputs=++|  OutDataType=sfix(16)  OutScaling=2^0  SaturateOnIntegerOverflow=on
  Sum2 : Sum  Inputs=|+-  OutDataType=sfix(16)  OutScaling=2^0  SaturateOnIntegerOverflow=on
  Tacho filter : TransferFcn  Numerator=0.03  Denominator="[8.475e-4  1]"
  Taco dynamics : TransferFcn  Numerator=1  Denominator="[1/(2014*2014)   2*0.294/2014  1]"
  Velocity gain : Gain  Orientation=down  Gain=0.03  ParameterDataType=sfix(16)  ParameterScaling=2^0  OutDataType=sfix(16)  OutScaling=2^0  SaturateOnIntegerOverflow=on  OutDataTypeStr=Inherit: Same as input  ParamDataTypeStr=Inherit: Same as input
  i_ref : Outport  OutDataType=sfix(16)  OutScaling=2^0
  wires:
  phi_ref/1 -> Sum/1
  Sum/1 -> Position gain/1
  Position gain/1 -> Sum1/2
  Velocity gain/1 -> Sum1/1
  Sum1/1 -> Sum2/1
  Sum2/1 -> Lead filter/1
  Rate controller/1 -> Sum2/2
  Taco dynamics/1 -> Rate controller/1
  Tacho filter/1 -> Taco dynamics/1
  Angular velocity/1 -> Tacho filter/1
  Lead filter/1 -> Integrator/1
  Integrator/1 -> i_ref/1
  w_ref/1 -> Velocity gain/1
  phi/1 -> Sum/2

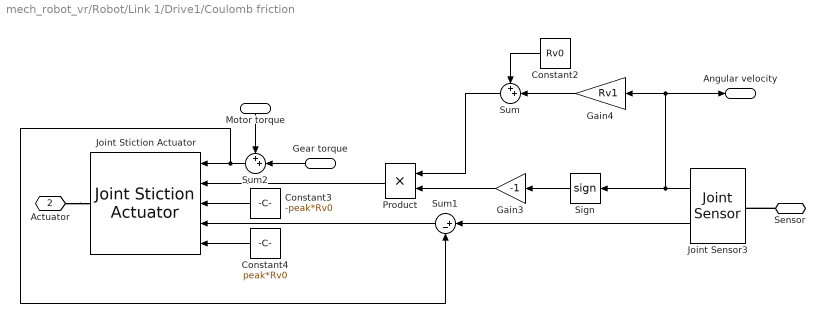
== system mech_robot_vr/Robot/Link 1/Drive1/Coulomb friction ==
  Motor torque : Inport  Orientation=down  OutDataType=sfix(16)  OutScaling=2^0
  Gear torque : Inport  Orientation=left  Port=2  OutDataType=sfix(16)  OutScaling=2^0
  Constant2 : Constant  Orientation=left  Value=Rv0  OutDataType=sfix(16)  OutScaling=2^0
  Constant3 : Constant  Orientation=left  Value=-peak*Rv0  OutDataType=sfix(16)  OutScaling=2^0
  Constant4 : Constant  Orientation=left  Value=peak*Rv0  OutDataType=sfix(16)  OutScaling=2^0
  Gain3 : Gain  Orientation=left  Gain=-1  ParameterDataType=sfix(16)  ParameterScaling=2^0  OutDataType=sfix(16)  OutScaling=2^0  SaturateOnIntegerOverflow=on  OutDataTypeStr=Inherit: Same as input  ParamDataTypeStr=Inherit: Same as input
  Gain4 : Gain  Orientation=left  Gain=Rv1  ParameterDataType=sfix(16)  ParameterScaling=2^0  OutDataType=sfix(16)  OutScaling=2^0  SaturateOnIntegerOverflow=on  OutDataTypeStr=Inherit: Same as input  ParamDataTypeStr=Inherit: Same as input
  Joint Sensor3 : mblibv1/Sensors &  Actuators/Joint Sensor  Description=Mechanical Blockset  Orientation=left  DialogController=MECH.DynMechDlgSource  SystemSampleTime=-1  PhysicalDomain=Mechanical  PortType=blob  Muxed=off  Pose=off  Angle=off  AngleUnits=rad  ArcVelocity=on  ArcVelocityUnits=rad/s  ArcAcceleration=off  ArcAccelerationUnits=deg/s^2  CoordPosition=off  CoordPositionUnits=m  Velocity=off  VelocityUnits=m/s  Acceleration=off  AccelerationUnits=m/s^2  Quaternion=off  QuaternionDT=off  QuaternionDDT=off  QuaternionUnits=off  OutputVector=[ 1 1 ]  ActiveIO=on  Width=2  DialogClass=MechanicalSensorBlock  Primitive=R1  Force=off  ForceUnits=N  Torque=on  TorqueUnits=N-m  ReferenceFrame=Absolute (INERTIAL)  ReactionSensedSide=Base  ReactionReferenceFrame=Absolute (World)  ReactionForce=off  ReactionForceUnits=N  ReactionMoment=off  ReactionMomentUnits=N-m
  Joint Stiction Actuator : mblibv1/Sensors &  Actuators/Joint Stiction Actuator  Description=Mechanical Blockset  Orientation=left  DialogController=MECH.DynMechDlgSource  SystemSampleTime=-1  PhysicalDomain=Mechanical  PortType=blob  ActuationStyle=Force  AngleUnits=deg  ArcVelocityUnits=deg/s  ArcAccelerationUnits=deg/s^2  CoordPositionUnits=m  VelocityUnits=m/s  AccelerationUnits=m/s^2  ForceUnits=N  TorqueUnits=N-m  ActiveIO=on  Width=5  DialogClass=EventActuatorBlock  Primitive=R1  FrictionalForceUnits=N  ExternalForceUnits=N  FrictionalTorqueUnits=N-m  ExternalTorqueUnits=N-m  LockingTolerance=1e-3
  Product : Product  Orientation=left  OutDataType=sfix(16)  OutScaling=2^0  SaturateOnIntegerOverflow=on  InputSameDT=on  OutDataTypeStr=Inherit: Same as first input
  Sign : Signum  Orientation=left
  Sum : Sum  Orientation=left  Inputs=++|  OutDataType=sfix(16)  OutScaling=2^0  SaturateOnIntegerOverflow=on  InputSameDT=on  OutDataTypeStr=Inherit: Same as first input
  Sum1 : Sum  Orientation=left  Inputs=|+-  OutDataType=sfix(16)  OutScaling=2^0  SaturateOnIntegerOverflow=on  InputSameDT=on  OutDataTypeStr=Inherit: Same as first input
  Sum2 : Sum  Orientation=left  Inputs=++|  OutDataType=sfix(16)  OutScaling=2^0  SaturateOnIntegerOverflow=on
  Sensor : PMIOPort  Orientation=left  Port=1  Side=Right
  Actuator : PMIOPort  Port=2  Side=Right
  Angular velocity : Outport  OutDataType=sfix(16)  OutScaling=2^0
  wires:
  Sum1/1 -> Joint Stiction Actuator/4
  Constant3/1 -> Joint Stiction Actuator/3
  Gain3/1 -> Product/2
  Constant2/1 -> Sum/1
  Gain4/1 -> Sum/2
  Constant4/1 -> Joint Stiction Actuator/5
  Joint Sensor3/2 -> Sum1/1
  Sum/1 -> Product/1
  Sign/1 -> Gain3/1
  Product/1 -> Joint Stiction Actuator/2
  Motor torque/1 -> Sum2/1
  Gear torque/1 -> Sum2/2
  Sum2/1 -> Joint Stiction Actuator/1, Sum1/2
  Joint Sensor3/1 -> Sign/1, Gain4/1, Angular velocity/1
  connections:
  Sensor/RConn1 -- Joint Sensor3/LConn1
  Actuator/RConn1 -- Joint Stiction Actuator/RConn1

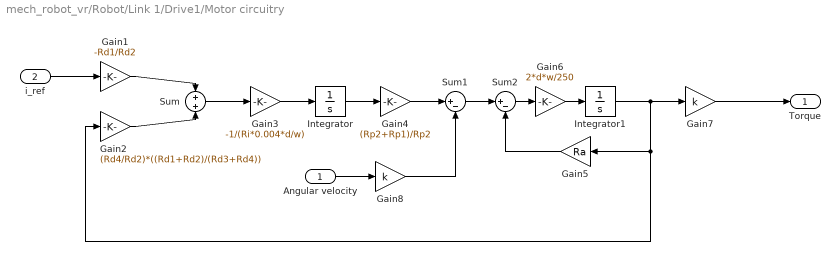
== system mech_robot_vr/Robot/Link 1/Drive1/Motor circuitry ==
  Angular velocity : Inport  OutDataType=sfix(16)  OutScaling=2^0
  i_ref : Inport  Port=2  OutDataType=sfix(16)  OutScaling=2^0
  Gain1 : Gain  Gain=-Rd1/Rd2  ParameterDataType=sfix(16)  ParameterScaling=2^0  OutDataType=sfix(16)  OutScaling=2^0  SaturateOnIntegerOverflow=on  OutDataTypeStr=Inherit: Same as input  ParamDataTypeStr=Inherit: Same as input
  Gain2 : Gain  Gain=(Rd4/Rd2)*((Rd1+Rd2)/(Rd3+Rd4))  ParameterDataType=sfix(16)  ParameterScaling=2^0  OutDataType=sfix(16)  OutScaling=2^0  SaturateOnIntegerOverflow=on  OutDataTypeStr=Inherit: Same as input  ParamDataTypeStr=Inherit: Same as input
  Gain3 : Gain  Gain=-1/(Ri*0.004*d/w)  ParameterDataType=sfix(16)  ParameterScaling=2^0  OutDataType=sfix(16)  OutScaling=2^0  SaturateOnIntegerOverflow=on  OutDataTypeStr=Inherit: Same as input  ParamDataTypeStr=Inherit: Same as input
  Gain4 : Gain  Gain=(Rp2+Rp1)/Rp2  ParameterDataType=sfix(16)  ParameterScaling=2^0  OutDataType=sfix(16)  OutScaling=2^0  SaturateOnIntegerOverflow=on  OutDataTypeStr=Inherit: Same as input  ParamDataTypeStr=Inherit: Same as input
  Gain5 : Gain  Orientation=left  Gain=Ra  ParameterDataType=sfix(16)  ParameterScaling=2^0  OutDataType=sfix(16)  OutScaling=2^0  SaturateOnIntegerOverflow=on  OutDataTypeStr=Inherit: Same as input  ParamDataTypeStr=Inherit: Same as input
  Gain6 : Gain  Gain=2*d*w/250  ParameterDataType=sfix(16)  ParameterScaling=2^0  OutDataType=sfix(16)  OutScaling=2^0  SaturateOnIntegerOverflow=on  OutDataTypeStr=Inherit: Same as input  ParamDataTypeStr=Inherit: Same as input
  Gain7 : Gain  Gain=k  ParameterDataType=sfix(16)  ParameterScaling=2^0  OutDataType=sfix(16)  OutScaling=2^0  SaturateOnIntegerOverflow=on  OutDataTypeStr=Inherit: Same as input  ParamDataTypeStr=Inherit: Same as input
  Gain8 : Gain  Gain=k  ParameterDataType=sfix(16)  ParameterScaling=2^0  OutDataType=sfix(16)  OutScaling=2^0  SaturateOnIntegerOverflow=on  OutDataTypeStr=Inherit: Same as input  ParamDataTypeStr=Inherit: Same as input
  Integrator : Integrator  ZeroCross=off
  Integrator1 : Integrator  ZeroCross=off
  Sum : Sum  OutDataType=sfix(16)  OutScaling=2^0  SaturateOnIntegerOverflow=on  InputSameDT=on  OutDataTypeStr=Inherit: Same as first input
  Sum1 : Sum  Inputs=|+-  OutDataType=sfix(16)  OutScaling=2^0  SaturateOnIntegerOverflow=on  InputSameDT=on  OutDataTypeStr=Inherit: Same as first input
  Sum2 : Sum  Inputs=|+-  OutDataType=sfix(16)  OutScaling=2^0  SaturateOnIntegerOverflow=on  InputSameDT=on  OutDataTypeStr=Inherit: Same as first input
  Torque : Outport  OutDataType=sfix(16)  OutScaling=2^0
  wires:
  Angular velocity/1 -> Gain8/1
  Gain8/1 -> Sum1/2
  Gain6/1 -> Integrator1/1
  Sum2/1 -> Gain6/1
  Gain5/1 -> Sum2/2
  Integrator1/1 -> Gain2/1, Gain5/1, Gain7/1
  Sum1/1 -> Sum2/1
  Gain4/1 -> Sum1/1
  Integrator/1 -> Gain4/1
  Gain3/1 -> Integrator/1
  Sum/1 -> Gain3/1
  Gain2/1 -> Sum/2
  Gain1/1 -> Sum/1
  i_ref/1 -> Gain1/1
  Gain7/1 -> Torque/1
